simulink model "lateral_autopilot_3f"  (R2016b)
settings: Solver=VariableStepAuto  StartTime=0.0  StopTime=t_end  RelTol=1e-3
values from neighbouring files (symbols this model uses):
  d = 2*deg2rad    [run_task_3f.m]
undefined symbols (not defined in the file or in its folder): A, B, C, D, delta_a_max, g, h, integrator_error_limit, k_d_phi, k_i_chi, k_i_phi, k_p_chi, k_p_phi, V_g, var_p, var_phi, var_r
settings Model: Creator=EllaLovise  LastModifiedBy=EllaLovise

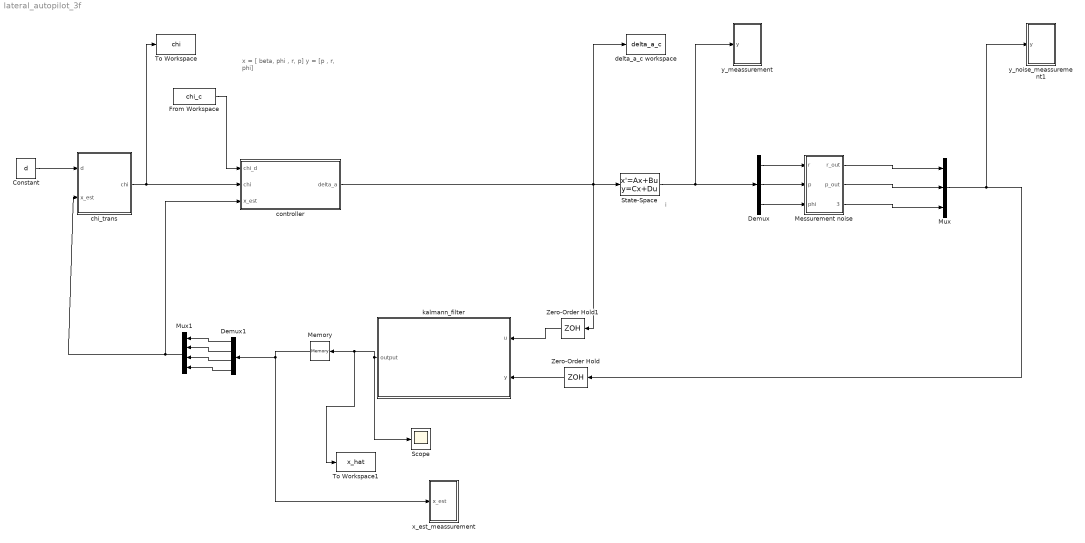
== system lateral_autopilot_3f ==
  note: x = [ beta, phi , r, p]
      | y = [p , r, phi]
  note: i
  Constant : Constant  Value=d
  Demux : Demux  Outputs=3
  Demux1 : Demux
  From Workspace : FromWorkspace  VariableName=chi_c  OutputAfterFinalValue=Holding final value
  Memory : Memory
  Messurement noise : Subsystem
  Mux : Mux  Inputs=3
  Mux1 : Mux
  Scope : Scope
  State-Space : StateSpace  A=A  B=B  C=C  D=D  X0=0
  To Workspace : ToWorkspace  VariableName=chi  SaveFormat=Structure With Time  SampleTime=-1
  To Workspace1 : ToWorkspace  VariableName=x_hat  SaveFormat=Structure With Time  SampleTime=-1
  Zero-Order Hold : ZeroOrderHold  SampleTime=h
  Zero-Order Hold1 : ZeroOrderHold  SampleTime=h
  chi_trans : Subsystem
  controller : Subsystem
  delta_a_c workspace : ToWorkspace  VariableName=delta_a_c  SaveFormat=Structure With Time  SampleTime=-1
  kalmann_filter : MATLAB Function  TreatAsAtomicUnit=on
  x_est_meassurement : Subsystem
  y_meassurement : Subsystem
  y_noise_meassurement1 : Subsystem
  wires:
  State-Space/1 -> Demux/1, y_meassurement/1(y)
  chi_trans/1(chi) -> To Workspace/1, controller/2("chi ")
  From Workspace/1 -> controller/1(chi_d)
  Zero-Order Hold/1 -> kalmann_filter/2(y)
  Zero-Order Hold1/1 -> kalmann_filter/1(u)
  controller/1(delta_a) -> delta_a_c workspace/1, State-Space/1, Zero-Order Hold1/1
  Demux/1 -> Messurement noise/1(r)
  Demux/2 -> Messurement noise/2(p)
  Messurement noise/1(r_out) -> Mux/1
  Messurement noise/2(p_out) -> Mux/2
  Demux/3 -> Messurement noise/3(phi)
  Mux/1 -> y_noise_meassurement1/1(y), Zero-Order Hold/1
  kalmann_filter/1(output) -> To Workspace1/1, Memory/1, Scope/1
  Messurement noise/3(phi_out) -> Mux/3
  Constant/1 -> chi_trans/1(d)
  Memory/1 -> x_est_meassurement/1(x_est), Demux1/1
  Demux1/1 -> Mux1/1
  Demux1/2 -> Mux1/2
  Demux1/4 -> Mux1/4
  Demux1/3 -> Mux1/3
  Mux1/1 -> controller/3(x_est), chi_trans/2(x_est)

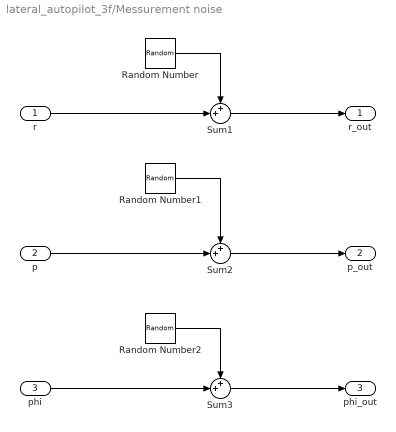
== system lateral_autopilot_3f/Messurement noise ==
  r : Inport
  p : Inport  Port=2
  phi : Inport  Port=3
  Random Number : RandomNumber  Variance=var_r
  Random Number1 : RandomNumber  Variance=var_p
  Random Number2 : RandomNumber  Variance=var_phi
  Sum1 : Sum  Inputs=++|
  Sum2 : Sum  Inputs=++|
  Sum3 : Sum  Inputs=++|
  r_out : Outport
  p_out : Outport  Port=2
  phi_out : Outport  Port=3
  wires:
  p/1 -> Sum2/2
  Sum1/1 -> r_out/1
  Sum2/1 -> p_out/1
  Sum3/1 -> phi_out/1
  Random Number/1 -> Sum1/1
  r/1 -> Sum1/2
  Random Number2/1 -> Sum3/1
  Random Number1/1 -> Sum2/1
  phi/1 -> Sum3/2

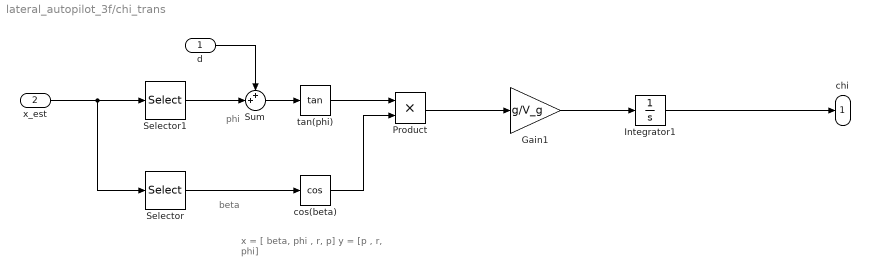
== system lateral_autopilot_3f/chi_trans ==
  note: phi
  note: x = [ beta, phi , r, p]
      | y = [p , r, phi]
  note: beta
  d : Inport
  x_est : Inport  Port=2
  Gain1 : Gain  Gain=g/V_g
  Integrator1 : Integrator
  Product : Product
  Selector : Selector  InputPortWidth=4  IndexOptions=Index vector (dialog)  Indices=[1]  OutputSizes=1
  Selector1 : Selector  InputPortWidth=4  IndexOptions=Index vector (dialog)  Indices=[2]  OutputSizes=1
  Sum : Sum  Inputs=++|
  cos(beta) : Trigonometry  Operator=cos
  tan(phi) : Trigonometry  Operator=tan
  chi : Outport
  wires:
  Integrator1/1 -> chi/1
  Gain1/1 -> Integrator1/1
  x_est/1 -> Selector/1, Selector1/1
  cos(beta)/1 -> Product/2
  tan(phi)/1 -> Product/1
  Selector/1 -> cos(beta)/1
  Product/1 -> Gain1/1
  Sum/1 -> tan(phi)/1
  Selector1/1 -> Sum/2
  d/1 -> Sum/1

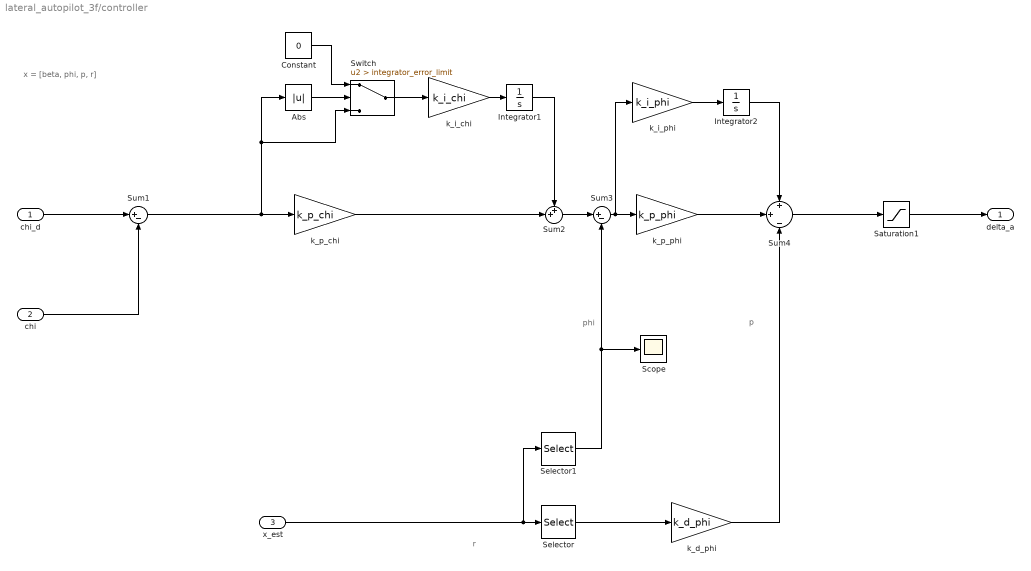
== system lateral_autopilot_3f/controller ==
  note: p
  note: phi
  note: r
  note: x = [beta, phi, p, r]
  chi_d : Inport
  "chi " : Inport  Port=2
  x_est : Inport  Port=3
  Abs : Abs
  Constant : Constant  Value=0
  Integrator1 : Integrator
  Integrator2 : Integrator
  Saturation1 : Saturate  UpperLimit=delta_a_max  LowerLimit=-1*delta_a_max
  Scope : Scope
  Selector : Selector  InputPortWidth=4  IndexOptions=Index vector (dialog)  Indices=[3]  OutputSizes=1
  Selector1 : Selector  InputPortWidth=4  IndexOptions=Index vector (dialog)  Indices=[2]  OutputSizes=1
  Sum1 : Sum  Inputs=|+-
  Sum2 : Sum  Inputs=++|
  Sum3 : Sum  Inputs=|+-
  Sum4 : Sum  Inputs=+|+|-
  Switch : Switch  Criteria=u2 > Threshold  Threshold=integrator_error_limit
  "k_d_phi " : Gain  Gain=k_d_phi
  k_i_chi : Gain  Gain=k_i_chi
  k_i_phi : Gain  Gain=k_i_phi
  k_p_chi : Gain  Gain=k_p_chi
  k_p_phi : Gain  Gain=k_p_phi
  delta_a : Outport
  wires:
  k_p_chi/1 -> Sum2/2
  Sum2/1 -> Sum3/1
  Sum3/1 -> k_p_phi/1, k_i_phi/1
  Integrator2/1 -> Sum4/1
  "k_d_phi "/1 -> Sum4/3
  k_p_phi/1 -> Sum4/2
  k_i_phi/1 -> Integrator2/1
  k_i_chi/1 -> Integrator1/1
  Integrator1/1 -> Sum2/1
  x_est/1 -> Selector1/1, Selector/1
  Sum1/1 -> Abs/1, Switch/3, k_p_chi/1
  "chi "/1 -> Sum1/2
  chi_d/1 -> Sum1/1
  Saturation1/1 -> delta_a/1
  Abs/1 -> Switch/2
  Switch/1 -> k_i_chi/1
  Constant/1 -> Switch/1
  Sum4/1 -> Saturation1/1
  Selector/1 -> "k_d_phi "/1
  Selector1/1 -> Scope/1, Sum3/2

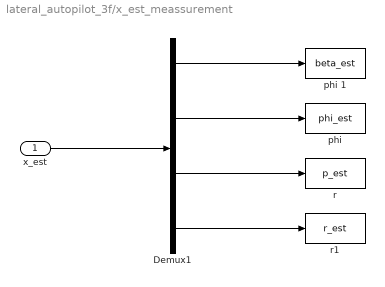
== system lateral_autopilot_3f/x_est_meassurement ==
  x_est : Inport
  Demux1 : Demux
  "phi " : ToWorkspace  VariableName=phi_est  SaveFormat=Structure With Time  SampleTime=-1
  phi 1 : ToWorkspace  VariableName=beta_est  SaveFormat=Structure With Time  SampleTime=-1
  r : ToWorkspace  VariableName=p_est  SaveFormat=Structure With Time  SampleTime=-1
  r1 : ToWorkspace  VariableName=r_est  SaveFormat=Structure With Time  SampleTime=-1
  wires:
  x_est/1 -> Demux1/1
  Demux1/2 -> "phi "/1
  Demux1/4 -> r1/1
  Demux1/3 -> r/1
  Demux1/1 -> phi 1/1

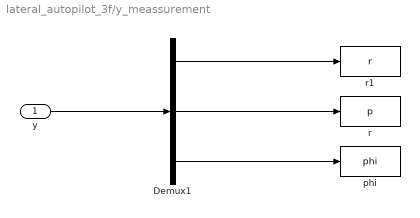
== system lateral_autopilot_3f/y_meassurement ==
  y : Inport
  Demux1 : Demux  Outputs=3
  "phi " : ToWorkspace  VariableName=phi  SaveFormat=Structure With Time  SampleTime=-1
  r : ToWorkspace  VariableName=p  SaveFormat=Structure With Time  SampleTime=-1
  r1 : ToWorkspace  VariableName=r  SaveFormat=Structure With Time  SampleTime=-1
  wires:
  y/1 -> Demux1/1
  Demux1/1 -> r1/1
  Demux1/2 -> r/1
  Demux1/3 -> "phi "/1

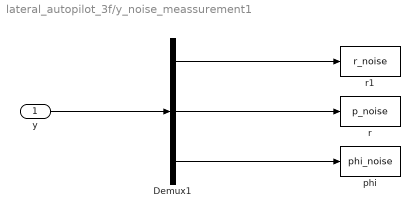
== system lateral_autopilot_3f/y_noise_meassurement1 ==
  y : Inport
  Demux1 : Demux  Outputs=3
  "phi " : ToWorkspace  VariableName=phi_noise  SaveFormat=Structure With Time  SampleTime=-1
  r : ToWorkspace  VariableName=p_noise  SaveFormat=Structure With Time  SampleTime=-1
  r1 : ToWorkspace  VariableName=r_noise  SaveFormat=Structure With Time  SampleTime=-1
  wires:
  y/1 -> Demux1/1
  Demux1/1 -> r1/1
  Demux1/2 -> r/1
  Demux1/3 -> "phi "/1

== matlab function lateral_autopilot_3f/kalmann_filter ==
  data: u input; y input; output output; system_information_struct parameter
function output = fcn(u,y, system_information_struct)
persistent P_priori init_flag x_priori

A_d = system_information_struct.A_d;
B_d = system_information_struct.B_d;
E_d = system_information_struct.E_d;
C_d = system_information_struct.C_d;
Q = system_information_struct.Q;
I = system_information_struct.I;
R = system_information_struct.R;

if isempty(init_flag) %check if first round 
    init_flag = 1;
    
    P_0_priori= eye(4); 
    x_0_priori = [0; 0; 0; 0];
    P_priori = P_0_priori;
    x_priori = x_0_priori;
end

% 1) Compute Kalman gain
L = P_priori * C_d' * inv( C_d * P_priori * C_d' + R); 

% 2) update error covariance matrix (corrector)
P_posteriori = ( I - L*C_d)*P_priori*( I- L*C_d)' + L* R*L';

% 3) Update estimate with measurement 
x_posteriori = x_priori + L * ( y - C_d*x_priori);

% 4) Project ahead (predictor)
x_next_priori = A_d * x_posteriori + B_d*u;
P_next_priori = A_d*P_posteriori*A_d'+ E_d*Q*E_d';

x_priori = x_next_priori;
P_priori = P_next_priori; 

output = x_posteriori;
